simulink model "SecRwLtStLgrstUpwdDnwdTrgtPosSelc"  (R2018b)
settings: Solver=FixedStepDiscrete  StartTime=0.0  StopTime=10.0  FixedStep=0.01  RelTol=1e-3
undefined symbols (not defined in the file or in its folder): KeSMSw4SAcsMd22SecRwLtStLegrstUpwdDnwdPos_Val, KeSMSw4SAcsMd22SecRwLtStLegrstUpwdDnwdPosMax_Val, KeSMSw4SAcsMd22SecRwLtStLegrstUpwdDnwdPosMin_Val, KeSMSw4SAcsMd26SecRwLtStLegrstUpwdDnwdPos_Val, KeSMSw4SAcsMd26SecRwLtStLegrstUpwdDnwdPosMax_Val, KeSMSw4SAcsMd26SecRwLtStLegrstUpwdDnwdPosMin_Val, KeSMSw4SLegrstCloseMdSecRwLtStLgrstUpwdDnwdPos_Val, KeSMSw4SLegrstCloseMdSecRwLtStLgrstUpwdDnwdPosMax_Val, KeSMSw4SLegrstCloseMdSecRwLtStLgrstUpwdDnwdPosMin_Val, KeSMSw4SLegrstOpenMdSecRwLtStLgrstUpwdDnwdPos_Val, KeSMSw4SLegrstOpenMdSecRwLtStLgrstUpwdDnwdPosMax_Val, KeSMSw4SLegrstOpenMdSecRwLtStLgrstUpwdDnwdPosMin_Val, KeSMSw4sLyingMDSecRwLtStLgrstUpwdDnwdPos_Val, KeSMSw4sLyingMDSecRwLtStLgrstUpwdDnwdPosMax_Val, KeSMSw4sLyingMDSecRwLtStLgrstUpwdDnwdPosMin_Val, KeSMSw4sRecoveryMDSecRwLtStLgrstUpwdDnwdPos_Val, KeSMSw4sRecoveryMDSecRwLtStLgrstUpwdDnwdPosMax_Val, KeSMSw4sRecoveryMDSecRwLtStLgrstUpwdDnwdPosMin_Val, KeSMSw4sVIPMDSecRwLtStLgrstUpwdDnwdPos_Val, KeSMSw4sVIPMDSecRwLtStLgrstUpwdDnwdPosMax_Val, KeSMSw4sVIPMDSecRwLtStLgrstUpwdDnwdPosMin_Val, KeSMSw6sAcsEntrySecRwLtStLgrstUpwdPos_Val, KeSMSw6sAcsEntrySecRwLtStLgrstUpwdPosMax_Val, KeSMSw6sAcsEntrySecRwLtStLgrstUpwdPosMin_Val, KeSMSw6sAcsExtSecRwLtStLgrstUpwdDnwdPos_Val, KeSMSw6sAcsExtSecRwLtStLgrstUpwdDnwdPosMax_Val, KeSMSw6sAcsExtSecRwLtStLgrstUpwdDnwdPosMin_Val, KeSMSw6sRecoveryMdSecRwLtStLgrstUpwdDnwdPos_Val, KeSMSw6sRecoveryMdSecRwLtStLgrstUpwdDnwdPosMax_Val, KeSMSw6sRecoveryMdSecRwLtStLgrstUpwdDnwdPosMin_Val, KeSMSw6sVIPSecRwLtStLgrstUpwdPos_Val, KeSMSw6sVIPSecRwLtStLgrstUpwdPosMax_Val, KeSMSw6sVIPSecRwLtStLgrstUpwdPosMin_Val, KeSMSwAcsEntrySecRwLtStLgrstUpwdPos_Val, KeSMSwAcsEntrySecRwLtStLgrstUpwdPosMax_Val, KeSMSwAcsEntrySecRwLtStLgrstUpwdPosMin_Val, KeSMSwAcsExtSecRwLtStLgrstUpwdDnwdPos_Val, KeSMSwAcsExtSecRwLtStLgrstUpwdDnwdPosMax_Val, KeSMSwAcsExtSecRwLtStLgrstUpwdDnwdPosMin_Val, KeSMSwAcsMd8SecRwLtStLgrstUpwdDnwdPos_Val, KeSMSwAcsMd8SecRwLtStLgrstUpwdDnwdPosMax_Val, KeSMSwAcsMd8SecRwLtStLgrstUpwdDnwdPosMin_Val, KeSMSwRecoveryMdSecRwLtStLgrstUpwdDnwdPos_Val, KeSMSwRecoveryMdSecRwLtStLgrstUpwdDnwdPosMax_Val, KeSMSwRecoveryMdSecRwLtStLgrstUpwdDnwdPosMin_Val, KeSMSwVIPSecRwLtStLgrstUpwdPos_Val, KeSMSwVIPSecRwLtStLgrstUpwdPosMax_Val, KeSMSwVIPSecRwLtStLgrstUpwdPosMin_Val
libraries: TrgtPosSelcLib x11
settings Model: Creator=sn2xws  LastModifiedBy=sn2xws
settings Model: ModifiedHistory=|
  | 2023.8.1 V2.0.0 CR401790 增加模式21-26
  | 2024.7.8 V3.0.0 557模式流程V1.9
settings DataIOCC: SaveFormat=StructureWithTime
settings OptimizationCC: DefaultParameterBehavior=Inlined  EnhancedBackFolding=on  PassReuseOutputArgsAs=Individual arguments  ZeroExternalMemoryAtStartup=off  ZeroInternalMemoryAtStartup=off  OptimizeBlockOrder=speed  DifferentSizesBufferReuse=on  OptimizationCustomize=off
settings DebuggingCC: ParameterTunabilityLossMsg=error
settings ModelReferenceCC: ModelReferenceNumInstancesAllowed=Single
settings SFSimCC: MATLABDynamicMemAlloc=off
settings RTWCC: SystemTargetFile=autosar.tlc  GenCodeOnly=on  TemplateMakefile=ert_default_tmf  Description=AUTOSAR  GenerateReport=on  IncludeHyperlinkInReport=on  LaunchReport=on  GenerateTraceInfo=on  GenerateTraceReport=on  GenerateTraceReportSl=on  GenerateTraceReportSf=on  GenerateTraceReportEml=on  GenerateCodeMetricsReport=on
settings CodeAppCC: ForceParamTrailComments=on  IgnoreCustomStorageClasses=off  OperatorAnnotations=on  SimulinkDataObjDesc=on  SFDataObjDesc=on  InsertBlockDesc=on
settings STFCustomTargetCC: TargetLangStandard=C99 (ISO)  MultiwordLength=256  ParMdlRefBuildCompliant=on  CompOptLevelCompliant=on  IncludeMdlTerminateFcn=off  CombineOutputUpdateFcns=on  SuppressErrorStatus=on  ERTCustomFileBanners=on  SupportNonFinite=off  SupportComplex=off  SupportContinuousTime=off  SupportNonInlinedSFcns=off  RemoveResetFunc=on  MATLABClassNameForMDSCustomization=Simulink.SoftwareTarget.ERTCustomization  AutosarCompliant=on  UseToolchainInfoCompliant=on  LookupTableObjectStructAxisOrder=2,1,3,4,...  LUTObjectStructOrderEvenSpacing=Size,Table,Breakpoints  SystemTargetFile=autosar.tlc
settings ERTTargetCC: TargetLangStandard=C99 (ISO)  ConcurrentExecutionCompliant=off  IncludeMdlTerminateFcn=off  SuppressErrorStatus=on  SupportNonFinite=off  SupportComplex=off  ModelStepFunctionPrototypeControlCompliant=off  CPPClassGenCompliant=off  AutosarCompliant=on  LookupTableObjectStructAxisOrder=2,1,3,4,...  LUTObjectStructOrderEvenSpacing=Size,Table,Breakpoints  InlinedParameterPlacement=NonHierarchical  ERTCustomFileTemplate=example_file_process.tlc  ERTFilePackagingFormat=Compact

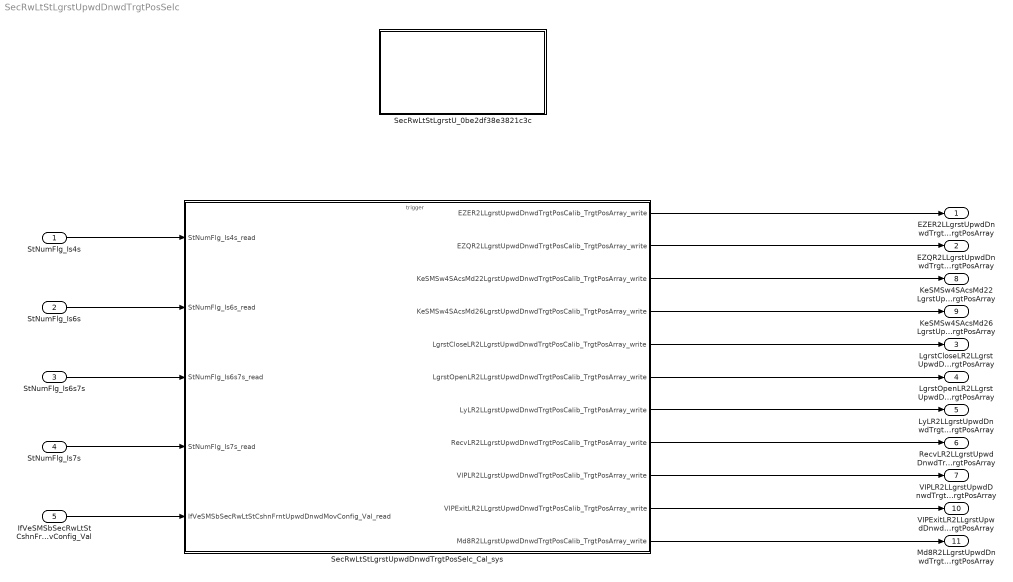
== system SecRwLtStLgrstUpwdDnwdTrgtPosSelc ==
  StNumFlg_Is4s : Inport  OutDataTypeStr=boolean  PortDimensions=1
  StNumFlg_Is6s : Inport  Port=2  OutDataTypeStr=boolean  PortDimensions=1
  StNumFlg_Is6s7s : Inport  Port=3  OutDataTypeStr=boolean  PortDimensions=1
  StNumFlg_Is7s : Inport  Port=4  OutDataTypeStr=boolean  PortDimensions=1
  IfVeSMSbSecRwLtStCshnFrntUpwdDnwdMovConfig_Val : Inport  Port=5  OutDataTypeStr=boolean  PortDimensions=1
  SecRwLtStLgrstU_0be2df38e3821c3c : Subsystem
  SecRwLtStLgrstUpwdDnwdTrgtPosSelc_Cal_sys : Subsystem
  EZER2LLgrstUpwdDnwdTrgtPosCalib_TrgtPosArray : Outport  Description=|  OutDataTypeStr=uint16  PortDimensions=3
      | 0:Pos
      | 1:Max
      | 2:Min
  EZQR2LLgrstUpwdDnwdTrgtPosCalib_TrgtPosArray : Outport  Description=|  Port=2  OutDataTypeStr=uint16  PortDimensions=3
      | 0:Pos
      | 1:Max
      | 2:Min
  LgrstCloseLR2LLgrstUpwdDnwdTrgtPosCalib_TrgtPosArray : Outport  Description=|  Port=3  OutDataTypeStr=uint16  PortDimensions=3
      | 0:Pos
      | 1:Max
      | 2:Min
  LgrstOpenLR2LLgrstUpwdDnwdTrgtPosCalib_TrgtPosArray : Outport  Description=|  Port=4  OutDataTypeStr=uint16  PortDimensions=3
      | 0:Pos
      | 1:Max
      | 2:Min
  LyLR2LLgrstUpwdDnwdTrgtPosCalib_TrgtPosArray : Outport  Description=|  Port=5  OutDataTypeStr=uint16  PortDimensions=3
      | 0:Pos
      | 1:Max
      | 2:Min
  RecvLR2LLgrstUpwdDnwdTrgtPosCalib_TrgtPosArray : Outport  Description=|  Port=6  OutDataTypeStr=uint16  PortDimensions=3
      | 0:Pos
      | 1:Max
      | 2:Min
  VIPLR2LLgrstUpwdDnwdTrgtPosCalib_TrgtPosArray : Outport  Description=|  Port=7  OutDataTypeStr=uint16  PortDimensions=3
      | 0:Pos
      | 1:Max
      | 2:Min
  KeSMSw4SAcsMd22LgrstUpwdDnwdTrgtPosCalib_TrgtPosArray : Outport  Description=|  Port=8  OutDataTypeStr=uint16  PortDimensions=3
      | 0:Pos
      | 1:Max
      | 2:Min
  KeSMSw4SAcsMd26LgrstUpwdDnwdTrgtPosCalib_TrgtPosArray : Outport  Description=|  Port=9  OutDataTypeStr=uint16  PortDimensions=3
      | 0:Pos
      | 1:Max
      | 2:Min
  VIPExitLR2LLgrstUpwdDnwdTrgtPosCalib_TrgtPosArray : Outport  Description=|  Port=10  OutDataTypeStr=uint16  PortDimensions=3
      | 0:Pos
      | 1:Max
      | 2:Min
  Md8R2LLgrstUpwdDnwdTrgtPosCalib_TrgtPosArray : Outport  Description=|  Port=11  OutDataTypeStr=uint16  PortDimensions=3
      | 0:Pos
      | 1:Max
      | 2:Min
  wires:
  StNumFlg_Is4s/1 -> SecRwLtStLgrstUpwdDnwdTrgtPosSelc_Cal_sys/1(StNumFlg_Is4s_read)
  StNumFlg_Is6s/1 -> SecRwLtStLgrstUpwdDnwdTrgtPosSelc_Cal_sys/2(StNumFlg_Is6s_read)
  StNumFlg_Is6s7s/1 -> SecRwLtStLgrstUpwdDnwdTrgtPosSelc_Cal_sys/3(StNumFlg_Is6s7s_read)
  StNumFlg_Is7s/1 -> SecRwLtStLgrstUpwdDnwdTrgtPosSelc_Cal_sys/4(StNumFlg_Is7s_read)
  SecRwLtStLgrstUpwdDnwdTrgtPosSelc_Cal_sys/1(EZER2LLgrstUpwdDnwdTrgtPosCalib_TrgtPosArray_write) -> EZER2LLgrstUpwdDnwdTrgtPosCalib_TrgtPosArray/1
  SecRwLtStLgrstUpwdDnwdTrgtPosSelc_Cal_sys/2(EZQR2LLgrstUpwdDnwdTrgtPosCalib_TrgtPosArray_write) -> EZQR2LLgrstUpwdDnwdTrgtPosCalib_TrgtPosArray/1
  SecRwLtStLgrstUpwdDnwdTrgtPosSelc_Cal_sys/5(LgrstCloseLR2LLgrstUpwdDnwdTrgtPosCalib_TrgtPosArray_write) -> LgrstCloseLR2LLgrstUpwdDnwdTrgtPosCalib_TrgtPosArray/1
  SecRwLtStLgrstUpwdDnwdTrgtPosSelc_Cal_sys/6(LgrstOpenLR2LLgrstUpwdDnwdTrgtPosCalib_TrgtPosArray_write) -> LgrstOpenLR2LLgrstUpwdDnwdTrgtPosCalib_TrgtPosArray/1
  SecRwLtStLgrstUpwdDnwdTrgtPosSelc_Cal_sys/7(LyLR2LLgrstUpwdDnwdTrgtPosCalib_TrgtPosArray_write) -> LyLR2LLgrstUpwdDnwdTrgtPosCalib_TrgtPosArray/1
  SecRwLtStLgrstUpwdDnwdTrgtPosSelc_Cal_sys/8(RecvLR2LLgrstUpwdDnwdTrgtPosCalib_TrgtPosArray_write) -> RecvLR2LLgrstUpwdDnwdTrgtPosCalib_TrgtPosArray/1
  SecRwLtStLgrstUpwdDnwdTrgtPosSelc_Cal_sys/9(VIPLR2LLgrstUpwdDnwdTrgtPosCalib_TrgtPosArray_write) -> VIPLR2LLgrstUpwdDnwdTrgtPosCalib_TrgtPosArray/1
  SecRwLtStLgrstUpwdDnwdTrgtPosSelc_Cal_sys/3(KeSMSw4SAcsMd22LgrstUpwdDnwdTrgtPosCalib_TrgtPosArray_write) -> KeSMSw4SAcsMd22LgrstUpwdDnwdTrgtPosCalib_TrgtPosArray/1
  SecRwLtStLgrstUpwdDnwdTrgtPosSelc_Cal_sys/4(KeSMSw4SAcsMd26LgrstUpwdDnwdTrgtPosCalib_TrgtPosArray_write) -> KeSMSw4SAcsMd26LgrstUpwdDnwdTrgtPosCalib_TrgtPosArray/1
  IfVeSMSbSecRwLtStCshnFrntUpwdDnwdMovConfig_Val/1 -> SecRwLtStLgrstUpwdDnwdTrgtPosSelc_Cal_sys/5(IfVeSMSbSecRwLtStCshnFrntUpwdDnwdMovConfig_Val_read)
  SecRwLtStLgrstUpwdDnwdTrgtPosSelc_Cal_sys/10(VIPExitLR2LLgrstUpwdDnwdTrgtPosCalib_TrgtPosArray_write) -> VIPExitLR2LLgrstUpwdDnwdTrgtPosCalib_TrgtPosArray/1
  SecRwLtStLgrstUpwdDnwdTrgtPosSelc_Cal_sys/11(Md8R2LLgrstUpwdDnwdTrgtPosCalib_TrgtPosArray_write) -> Md8R2LLgrstUpwdDnwdTrgtPosCalib_TrgtPosArray/1

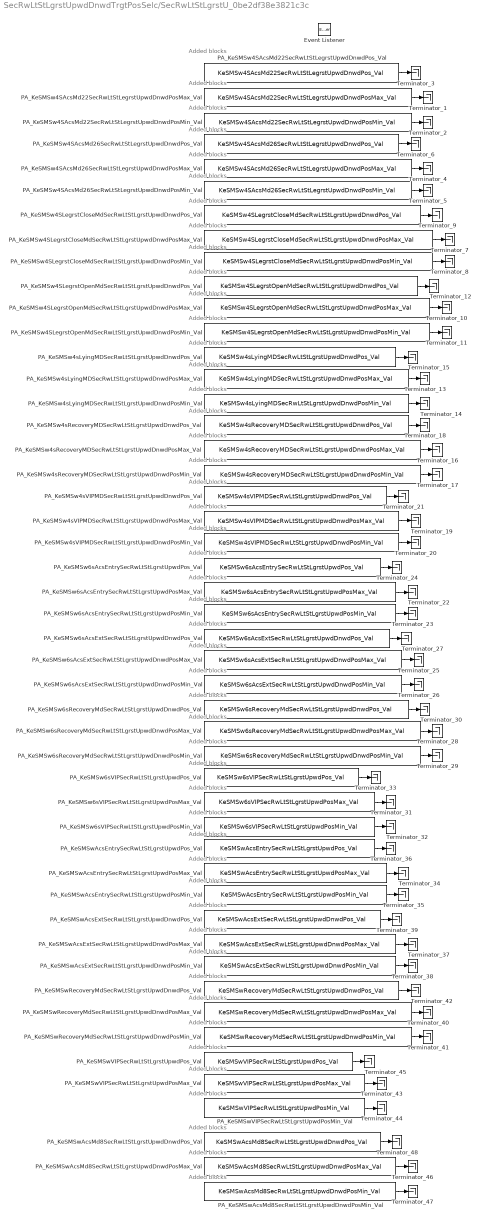
== system SecRwLtStLgrstUpwdDnwdTrgtPosSelc/SecRwLtStLgrstU_0be2df38e3821c3c ==
  note: Added blocks
  note: Added blocks
  note: Added blocks
  note: Added blocks
  note: Added blocks
  note: Added blocks
  note: Added blocks
  note: Added blocks
  note: Added blocks
  note: Added blocks
  note: Added blocks
  note: Added blocks
  note: Added blocks
  note: Added blocks
  note: Added blocks
  note: Added blocks
  note: Added blocks
  note: Added blocks
  note: Added blocks
  note: Added blocks
  note: Added blocks
  note: Added blocks
  note: Added blocks
  note: Added blocks
  note: Added blocks
  note: Added blocks
  note: Added blocks
  note: Added blocks
  note: Added blocks
  note: Added blocks
  note: Added blocks
  note: Added blocks
  note: Added blocks
  note: Added blocks
  note: Added blocks
  note: Added blocks
  note: Added blocks
  note: Added blocks
  note: Added blocks
  note: Added blocks
  note: Added blocks
  note: Added blocks
  note: Added blocks
  note: Added blocks
  note: Added blocks
  note: Added blocks
  note: Added blocks
  note: Added blocks
  Event Listener : EventListener  EventName=reset
  PA_KeSMSw4SAcsMd22SecRwLtStLegrstUpwdDnwdPosMax_Val : Constant  Value=KeSMSw4SAcsMd22SecRwLtStLegrstUpwdDnwdPosMax_Val
  PA_KeSMSw4SAcsMd22SecRwLtStLegrstUpwdDnwdPosMin_Val : Constant  Value=KeSMSw4SAcsMd22SecRwLtStLegrstUpwdDnwdPosMin_Val
  PA_KeSMSw4SAcsMd22SecRwLtStLegrstUpwdDnwdPos_Val : Constant  Value=KeSMSw4SAcsMd22SecRwLtStLegrstUpwdDnwdPos_Val
  PA_KeSMSw4SAcsMd26SecRwLtStLegrstUpwdDnwdPosMax_Val : Constant  Value=KeSMSw4SAcsMd26SecRwLtStLegrstUpwdDnwdPosMax_Val
  PA_KeSMSw4SAcsMd26SecRwLtStLegrstUpwdDnwdPosMin_Val : Constant  Value=KeSMSw4SAcsMd26SecRwLtStLegrstUpwdDnwdPosMin_Val
  PA_KeSMSw4SAcsMd26SecRwLtStLegrstUpwdDnwdPos_Val : Constant  Value=KeSMSw4SAcsMd26SecRwLtStLegrstUpwdDnwdPos_Val
  PA_KeSMSw4SLegrstCloseMdSecRwLtStLgrstUpwdDnwdPosMax_Val : Constant  Value=KeSMSw4SLegrstCloseMdSecRwLtStLgrstUpwdDnwdPosMax_Val
  PA_KeSMSw4SLegrstCloseMdSecRwLtStLgrstUpwdDnwdPosMin_Val : Constant  Value=KeSMSw4SLegrstCloseMdSecRwLtStLgrstUpwdDnwdPosMin_Val
  PA_KeSMSw4SLegrstCloseMdSecRwLtStLgrstUpwdDnwdPos_Val : Constant  Value=KeSMSw4SLegrstCloseMdSecRwLtStLgrstUpwdDnwdPos_Val
  PA_KeSMSw4SLegrstOpenMdSecRwLtStLgrstUpwdDnwdPosMax_Val : Constant  Value=KeSMSw4SLegrstOpenMdSecRwLtStLgrstUpwdDnwdPosMax_Val
  PA_KeSMSw4SLegrstOpenMdSecRwLtStLgrstUpwdDnwdPosMin_Val : Constant  Value=KeSMSw4SLegrstOpenMdSecRwLtStLgrstUpwdDnwdPosMin_Val
  PA_KeSMSw4SLegrstOpenMdSecRwLtStLgrstUpwdDnwdPos_Val : Constant  Value=KeSMSw4SLegrstOpenMdSecRwLtStLgrstUpwdDnwdPos_Val
  PA_KeSMSw4sLyingMDSecRwLtStLgrstUpwdDnwdPosMax_Val : Constant  Value=KeSMSw4sLyingMDSecRwLtStLgrstUpwdDnwdPosMax_Val
  PA_KeSMSw4sLyingMDSecRwLtStLgrstUpwdDnwdPosMin_Val : Constant  Value=KeSMSw4sLyingMDSecRwLtStLgrstUpwdDnwdPosMin_Val
  PA_KeSMSw4sLyingMDSecRwLtStLgrstUpwdDnwdPos_Val : Constant  Value=KeSMSw4sLyingMDSecRwLtStLgrstUpwdDnwdPos_Val
  PA_KeSMSw4sRecoveryMDSecRwLtStLgrstUpwdDnwdPosMax_Val : Constant  Value=KeSMSw4sRecoveryMDSecRwLtStLgrstUpwdDnwdPosMax_Val
  PA_KeSMSw4sRecoveryMDSecRwLtStLgrstUpwdDnwdPosMin_Val : Constant  Value=KeSMSw4sRecoveryMDSecRwLtStLgrstUpwdDnwdPosMin_Val
  PA_KeSMSw4sRecoveryMDSecRwLtStLgrstUpwdDnwdPos_Val : Constant  Value=KeSMSw4sRecoveryMDSecRwLtStLgrstUpwdDnwdPos_Val
  PA_KeSMSw4sVIPMDSecRwLtStLgrstUpwdDnwdPosMax_Val : Constant  Value=KeSMSw4sVIPMDSecRwLtStLgrstUpwdDnwdPosMax_Val
  PA_KeSMSw4sVIPMDSecRwLtStLgrstUpwdDnwdPosMin_Val : Constant  Value=KeSMSw4sVIPMDSecRwLtStLgrstUpwdDnwdPosMin_Val
  PA_KeSMSw4sVIPMDSecRwLtStLgrstUpwdDnwdPos_Val : Constant  Value=KeSMSw4sVIPMDSecRwLtStLgrstUpwdDnwdPos_Val
  PA_KeSMSw6sAcsEntrySecRwLtStLgrstUpwdPosMax_Val : Constant  Value=KeSMSw6sAcsEntrySecRwLtStLgrstUpwdPosMax_Val
  PA_KeSMSw6sAcsEntrySecRwLtStLgrstUpwdPosMin_Val : Constant  Value=KeSMSw6sAcsEntrySecRwLtStLgrstUpwdPosMin_Val
  PA_KeSMSw6sAcsEntrySecRwLtStLgrstUpwdPos_Val : Constant  Value=KeSMSw6sAcsEntrySecRwLtStLgrstUpwdPos_Val
  PA_KeSMSw6sAcsExtSecRwLtStLgrstUpwdDnwdPosMax_Val : Constant  Value=KeSMSw6sAcsExtSecRwLtStLgrstUpwdDnwdPosMax_Val
  PA_KeSMSw6sAcsExtSecRwLtStLgrstUpwdDnwdPosMin_Val : Constant  Value=KeSMSw6sAcsExtSecRwLtStLgrstUpwdDnwdPosMin_Val
  PA_KeSMSw6sAcsExtSecRwLtStLgrstUpwdDnwdPos_Val : Constant  Value=KeSMSw6sAcsExtSecRwLtStLgrstUpwdDnwdPos_Val
  PA_KeSMSw6sRecoveryMdSecRwLtStLgrstUpwdDnwdPosMax_Val : Constant  Value=KeSMSw6sRecoveryMdSecRwLtStLgrstUpwdDnwdPosMax_Val
  PA_KeSMSw6sRecoveryMdSecRwLtStLgrstUpwdDnwdPosMin_Val : Constant  Value=KeSMSw6sRecoveryMdSecRwLtStLgrstUpwdDnwdPosMin_Val
  PA_KeSMSw6sRecoveryMdSecRwLtStLgrstUpwdDnwdPos_Val : Constant  Value=KeSMSw6sRecoveryMdSecRwLtStLgrstUpwdDnwdPos_Val
  PA_KeSMSw6sVIPSecRwLtStLgrstUpwdPosMax_Val : Constant  Value=KeSMSw6sVIPSecRwLtStLgrstUpwdPosMax_Val
  PA_KeSMSw6sVIPSecRwLtStLgrstUpwdPosMin_Val : Constant  Value=KeSMSw6sVIPSecRwLtStLgrstUpwdPosMin_Val
  PA_KeSMSw6sVIPSecRwLtStLgrstUpwdPos_Val : Constant  Value=KeSMSw6sVIPSecRwLtStLgrstUpwdPos_Val
  PA_KeSMSwAcsEntrySecRwLtStLgrstUpwdPosMax_Val : Constant  Value=KeSMSwAcsEntrySecRwLtStLgrstUpwdPosMax_Val
  PA_KeSMSwAcsEntrySecRwLtStLgrstUpwdPosMin_Val : Constant  Value=KeSMSwAcsEntrySecRwLtStLgrstUpwdPosMin_Val
  PA_KeSMSwAcsEntrySecRwLtStLgrstUpwdPos_Val : Constant  Value=KeSMSwAcsEntrySecRwLtStLgrstUpwdPos_Val
  PA_KeSMSwAcsExtSecRwLtStLgrstUpwdDnwdPosMax_Val : Constant  Value=KeSMSwAcsExtSecRwLtStLgrstUpwdDnwdPosMax_Val
  PA_KeSMSwAcsExtSecRwLtStLgrstUpwdDnwdPosMin_Val : Constant  Value=KeSMSwAcsExtSecRwLtStLgrstUpwdDnwdPosMin_Val
  PA_KeSMSwAcsExtSecRwLtStLgrstUpwdDnwdPos_Val : Constant  Value=KeSMSwAcsExtSecRwLtStLgrstUpwdDnwdPos_Val
  PA_KeSMSwAcsMd8SecRwLtStLgrstUpwdDnwdPosMax_Val : Constant  Value=KeSMSwAcsMd8SecRwLtStLgrstUpwdDnwdPosMax_Val
  PA_KeSMSwAcsMd8SecRwLtStLgrstUpwdDnwdPosMin_Val : Constant  Value=KeSMSwAcsMd8SecRwLtStLgrstUpwdDnwdPosMin_Val
  PA_KeSMSwAcsMd8SecRwLtStLgrstUpwdDnwdPos_Val : Constant  Value=KeSMSwAcsMd8SecRwLtStLgrstUpwdDnwdPos_Val
  PA_KeSMSwRecoveryMdSecRwLtStLgrstUpwdDnwdPosMax_Val : Constant  Value=KeSMSwRecoveryMdSecRwLtStLgrstUpwdDnwdPosMax_Val
  PA_KeSMSwRecoveryMdSecRwLtStLgrstUpwdDnwdPosMin_Val : Constant  Value=KeSMSwRecoveryMdSecRwLtStLgrstUpwdDnwdPosMin_Val
  PA_KeSMSwRecoveryMdSecRwLtStLgrstUpwdDnwdPos_Val : Constant  Value=KeSMSwRecoveryMdSecRwLtStLgrstUpwdDnwdPos_Val
  PA_KeSMSwVIPSecRwLtStLgrstUpwdPosMax_Val : Constant  Value=KeSMSwVIPSecRwLtStLgrstUpwdPosMax_Val
  PA_KeSMSwVIPSecRwLtStLgrstUpwdPosMin_Val : Constant  Value=KeSMSwVIPSecRwLtStLgrstUpwdPosMin_Val
  PA_KeSMSwVIPSecRwLtStLgrstUpwdPos_Val : Constant  Value=KeSMSwVIPSecRwLtStLgrstUpwdPos_Val
  Terminator_{1..48} (48 alike) : Terminator
  wires:
  PA_KeSMSw4SAcsMd22SecRwLtStLegrstUpwdDnwdPosMax_Val/1 -> Terminator_1/1
  PA_KeSMSw4SAcsMd22SecRwLtStLegrstUpwdDnwdPosMin_Val/1 -> Terminator_2/1
  PA_KeSMSw4SAcsMd22SecRwLtStLegrstUpwdDnwdPos_Val/1 -> Terminator_3/1
  PA_KeSMSw4SAcsMd26SecRwLtStLegrstUpwdDnwdPosMax_Val/1 -> Terminator_4/1
  PA_KeSMSw4SAcsMd26SecRwLtStLegrstUpwdDnwdPosMin_Val/1 -> Terminator_5/1
  PA_KeSMSw4SAcsMd26SecRwLtStLegrstUpwdDnwdPos_Val/1 -> Terminator_6/1
  PA_KeSMSw4SLegrstCloseMdSecRwLtStLgrstUpwdDnwdPosMax_Val/1 -> Terminator_7/1
  PA_KeSMSw4SLegrstCloseMdSecRwLtStLgrstUpwdDnwdPosMin_Val/1 -> Terminator_8/1
  PA_KeSMSw4SLegrstCloseMdSecRwLtStLgrstUpwdDnwdPos_Val/1 -> Terminator_9/1
  PA_KeSMSw4SLegrstOpenMdSecRwLtStLgrstUpwdDnwdPosMax_Val/1 -> Terminator_10/1
  PA_KeSMSw4SLegrstOpenMdSecRwLtStLgrstUpwdDnwdPosMin_Val/1 -> Terminator_11/1
  PA_KeSMSw4SLegrstOpenMdSecRwLtStLgrstUpwdDnwdPos_Val/1 -> Terminator_12/1
  PA_KeSMSw4sLyingMDSecRwLtStLgrstUpwdDnwdPosMax_Val/1 -> Terminator_13/1
  PA_KeSMSw4sLyingMDSecRwLtStLgrstUpwdDnwdPosMin_Val/1 -> Terminator_14/1
  PA_KeSMSw4sLyingMDSecRwLtStLgrstUpwdDnwdPos_Val/1 -> Terminator_15/1
  PA_KeSMSw4sRecoveryMDSecRwLtStLgrstUpwdDnwdPosMax_Val/1 -> Terminator_16/1
  PA_KeSMSw4sRecoveryMDSecRwLtStLgrstUpwdDnwdPosMin_Val/1 -> Terminator_17/1
  PA_KeSMSw4sRecoveryMDSecRwLtStLgrstUpwdDnwdPos_Val/1 -> Terminator_18/1
  PA_KeSMSw4sVIPMDSecRwLtStLgrstUpwdDnwdPosMax_Val/1 -> Terminator_19/1
  PA_KeSMSw4sVIPMDSecRwLtStLgrstUpwdDnwdPosMin_Val/1 -> Terminator_20/1
  PA_KeSMSw4sVIPMDSecRwLtStLgrstUpwdDnwdPos_Val/1 -> Terminator_21/1
  PA_KeSMSw6sAcsEntrySecRwLtStLgrstUpwdPosMax_Val/1 -> Terminator_22/1
  PA_KeSMSw6sAcsEntrySecRwLtStLgrstUpwdPosMin_Val/1 -> Terminator_23/1
  PA_KeSMSw6sAcsEntrySecRwLtStLgrstUpwdPos_Val/1 -> Terminator_24/1
  PA_KeSMSw6sAcsExtSecRwLtStLgrstUpwdDnwdPosMax_Val/1 -> Terminator_25/1
  PA_KeSMSw6sAcsExtSecRwLtStLgrstUpwdDnwdPosMin_Val/1 -> Terminator_26/1
  PA_KeSMSw6sAcsExtSecRwLtStLgrstUpwdDnwdPos_Val/1 -> Terminator_27/1
  PA_KeSMSw6sRecoveryMdSecRwLtStLgrstUpwdDnwdPosMax_Val/1 -> Terminator_28/1
  PA_KeSMSw6sRecoveryMdSecRwLtStLgrstUpwdDnwdPosMin_Val/1 -> Terminator_29/1
  PA_KeSMSw6sRecoveryMdSecRwLtStLgrstUpwdDnwdPos_Val/1 -> Terminator_30/1
  PA_KeSMSw6sVIPSecRwLtStLgrstUpwdPosMax_Val/1 -> Terminator_31/1
  PA_KeSMSw6sVIPSecRwLtStLgrstUpwdPosMin_Val/1 -> Terminator_32/1
  PA_KeSMSw6sVIPSecRwLtStLgrstUpwdPos_Val/1 -> Terminator_33/1
  PA_KeSMSwAcsEntrySecRwLtStLgrstUpwdPosMax_Val/1 -> Terminator_34/1
  PA_KeSMSwAcsEntrySecRwLtStLgrstUpwdPosMin_Val/1 -> Terminator_35/1
  PA_KeSMSwAcsEntrySecRwLtStLgrstUpwdPos_Val/1 -> Terminator_36/1
  PA_KeSMSwAcsExtSecRwLtStLgrstUpwdDnwdPosMax_Val/1 -> Terminator_37/1
  PA_KeSMSwAcsExtSecRwLtStLgrstUpwdDnwdPosMin_Val/1 -> Terminator_38/1
  PA_KeSMSwAcsExtSecRwLtStLgrstUpwdDnwdPos_Val/1 -> Terminator_39/1
  PA_KeSMSwRecoveryMdSecRwLtStLgrstUpwdDnwdPosMax_Val/1 -> Terminator_40/1
  PA_KeSMSwRecoveryMdSecRwLtStLgrstUpwdDnwdPosMin_Val/1 -> Terminator_41/1
  PA_KeSMSwRecoveryMdSecRwLtStLgrstUpwdDnwdPos_Val/1 -> Terminator_42/1
  PA_KeSMSwVIPSecRwLtStLgrstUpwdPosMax_Val/1 -> Terminator_43/1
  PA_KeSMSwVIPSecRwLtStLgrstUpwdPosMin_Val/1 -> Terminator_44/1
  PA_KeSMSwVIPSecRwLtStLgrstUpwdPos_Val/1 -> Terminator_45/1
  PA_KeSMSwAcsMd8SecRwLtStLgrstUpwdDnwdPosMax_Val/1 -> Terminator_46/1
  PA_KeSMSwAcsMd8SecRwLtStLgrstUpwdDnwdPosMin_Val/1 -> Terminator_47/1
  PA_KeSMSwAcsMd8SecRwLtStLgrstUpwdDnwdPos_Val/1 -> Terminator_48/1

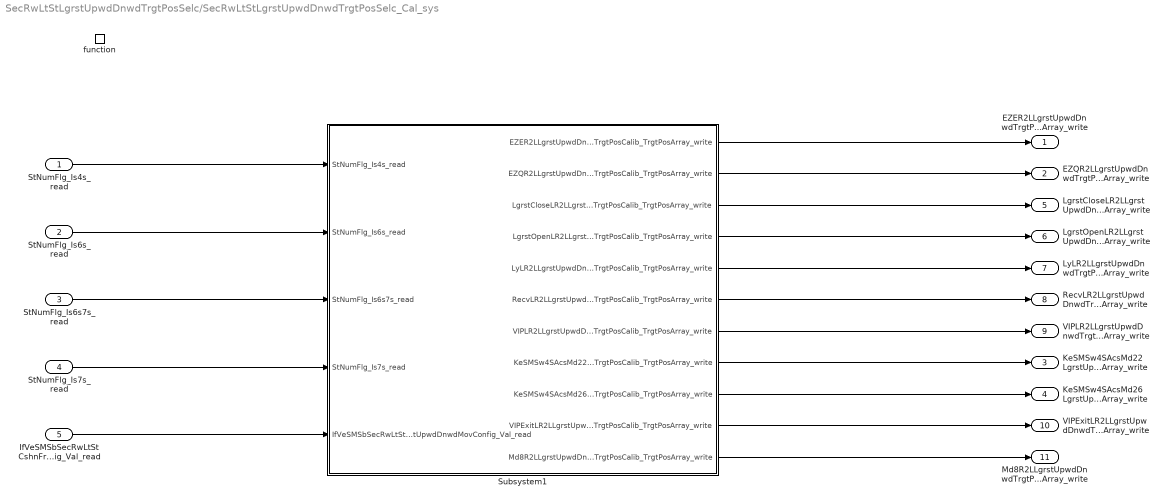
== system SecRwLtStLgrstUpwdDnwdTrgtPosSelc/SecRwLtStLgrstUpwdDnwdTrgtPosSelc_Cal_sys ==
  StNumFlg_Is4s_read : Inport
  StNumFlg_Is6s_read : Inport  Port=2
  StNumFlg_Is6s7s_read : Inport  Port=3
  StNumFlg_Is7s_read : Inport  Port=4
  IfVeSMSbSecRwLtStCshnFrntUpwdDnwdMovConfig_Val_read : Inport  Port=5
  function : TriggerPort  TriggerType=function-call  IsSimulinkFunction=on  FunctionName=SecRwLtStLgrstUpwdDnwdTrgtPosSelc_Cal  VariantControl=(inherit)
  Subsystem1 : Subsystem
  EZER2LLgrstUpwdDnwdTrgtPosCalib_TrgtPosArray_write : Outport
      settings: EnsureOutportIsVirtual=on
  EZQR2LLgrstUpwdDnwdTrgtPosCalib_TrgtPosArray_write : Outport  Port=2
      settings: EnsureOutportIsVirtual=on
  KeSMSw4SAcsMd22LgrstUpwdDnwdTrgtPosCalib_TrgtPosArray_write : Outport  Port=3
      settings: EnsureOutportIsVirtual=on
  KeSMSw4SAcsMd26LgrstUpwdDnwdTrgtPosCalib_TrgtPosArray_write : Outport  Port=4
      settings: EnsureOutportIsVirtual=on
  LgrstCloseLR2LLgrstUpwdDnwdTrgtPosCalib_TrgtPosArray_write : Outport  Port=5
      settings: EnsureOutportIsVirtual=on
  LgrstOpenLR2LLgrstUpwdDnwdTrgtPosCalib_TrgtPosArray_write : Outport  Port=6
      settings: EnsureOutportIsVirtual=on
  LyLR2LLgrstUpwdDnwdTrgtPosCalib_TrgtPosArray_write : Outport  Port=7
      settings: EnsureOutportIsVirtual=on
  RecvLR2LLgrstUpwdDnwdTrgtPosCalib_TrgtPosArray_write : Outport  Port=8
      settings: EnsureOutportIsVirtual=on
  VIPLR2LLgrstUpwdDnwdTrgtPosCalib_TrgtPosArray_write : Outport  Port=9
      settings: EnsureOutportIsVirtual=on
  VIPExitLR2LLgrstUpwdDnwdTrgtPosCalib_TrgtPosArray_write : Outport  Port=10
      settings: EnsureOutportIsVirtual=on
  Md8R2LLgrstUpwdDnwdTrgtPosCalib_TrgtPosArray_write : Outport  Port=11
      settings: EnsureOutportIsVirtual=on
  wires:
  Subsystem1/3(LgrstCloseLR2LLgrstUpwdDnwdTrgtPosCalib_TrgtPosArray_write) -> LgrstCloseLR2LLgrstUpwdDnwdTrgtPosCalib_TrgtPosArray_write/1
  Subsystem1/4(LgrstOpenLR2LLgrstUpwdDnwdTrgtPosCalib_TrgtPosArray_write) -> LgrstOpenLR2LLgrstUpwdDnwdTrgtPosCalib_TrgtPosArray_write/1
  Subsystem1/5(LyLR2LLgrstUpwdDnwdTrgtPosCalib_TrgtPosArray_write) -> LyLR2LLgrstUpwdDnwdTrgtPosCalib_TrgtPosArray_write/1
  Subsystem1/6(RecvLR2LLgrstUpwdDnwdTrgtPosCalib_TrgtPosArray_write) -> RecvLR2LLgrstUpwdDnwdTrgtPosCalib_TrgtPosArray_write/1
  Subsystem1/7(VIPLR2LLgrstUpwdDnwdTrgtPosCalib_TrgtPosArray_write) -> VIPLR2LLgrstUpwdDnwdTrgtPosCalib_TrgtPosArray_write/1
  Subsystem1/1(EZER2LLgrstUpwdDnwdTrgtPosCalib_TrgtPosArray_write) -> EZER2LLgrstUpwdDnwdTrgtPosCalib_TrgtPosArray_write/1
  Subsystem1/2(EZQR2LLgrstUpwdDnwdTrgtPosCalib_TrgtPosArray_write) -> EZQR2LLgrstUpwdDnwdTrgtPosCalib_TrgtPosArray_write/1
  Subsystem1/8(KeSMSw4SAcsMd22LgrstUpwdDnwdTrgtPosCalib_TrgtPosArray_write) -> KeSMSw4SAcsMd22LgrstUpwdDnwdTrgtPosCalib_TrgtPosArray_write/1
  Subsystem1/9(KeSMSw4SAcsMd26LgrstUpwdDnwdTrgtPosCalib_TrgtPosArray_write) -> KeSMSw4SAcsMd26LgrstUpwdDnwdTrgtPosCalib_TrgtPosArray_write/1
  StNumFlg_Is4s_read/1 -> Subsystem1/1(StNumFlg_Is4s_read)
  StNumFlg_Is6s_read/1 -> Subsystem1/2(StNumFlg_Is6s_read)
  StNumFlg_Is6s7s_read/1 -> Subsystem1/3(StNumFlg_Is6s7s_read)
  StNumFlg_Is7s_read/1 -> Subsystem1/4(StNumFlg_Is7s_read)
  IfVeSMSbSecRwLtStCshnFrntUpwdDnwdMovConfig_Val_read/1 -> Subsystem1/5(IfVeSMSbSecRwLtStCshnFrntUpwdDnwdMovConfig_Val_read)
  Subsystem1/10(VIPExitLR2LLgrstUpwdDnwdTrgtPosCalib_TrgtPosArray_write) -> VIPExitLR2LLgrstUpwdDnwdTrgtPosCalib_TrgtPosArray_write/1
  Subsystem1/11(Md8R2LLgrstUpwdDnwdTrgtPosCalib_TrgtPosArray_write) -> Md8R2LLgrstUpwdDnwdTrgtPosCalib_TrgtPosArray_write/1

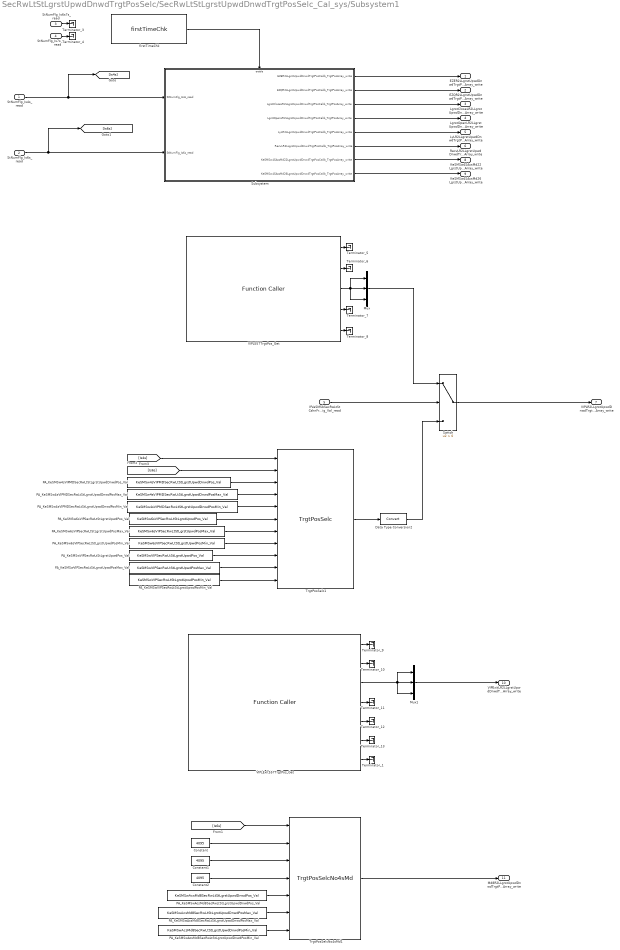
== system SecRwLtStLgrstUpwdDnwdTrgtPosSelc/SecRwLtStLgrstUpwdDnwdTrgtPosSelc_Cal_sys/Subsystem1 ==
  StNumFlg_Is4s_read : Inport
  StNumFlg_Is6s_read : Inport  Port=2
  StNumFlg_Is6s7s_read : Inport  Port=3
  StNumFlg_Is7s_read : Inport  Port=4
  IfVeSMSbSecRwLtStCshnFrntUpwdDnwdMovConfig_Val_read : Inport  Port=5
  Constant : Constant  Value=4095  OutDataTypeStr=uint16
  Constant1 : Constant  Value=4095  OutDataTypeStr=uint16
  Constant2 : Constant  Value=4095  OutDataTypeStr=uint16
  Data Type Conversion2 : DataTypeConversion
  Mux : Mux  Inputs=3
  Mux1 : Mux  Inputs=3
  PA_KeSMSw4sVIPMDSecRwLtStLgrstUpwdDnwdPosMax_Val : Constant  Value=KeSMSw4sVIPMDSecRwLtStLgrstUpwdDnwdPosMax_Val
  PA_KeSMSw4sVIPMDSecRwLtStLgrstUpwdDnwdPosMin_Val : Constant  Value=KeSMSw4sVIPMDSecRwLtStLgrstUpwdDnwdPosMin_Val
  PA_KeSMSw4sVIPMDSecRwLtStLgrstUpwdDnwdPos_Val : Constant  Value=KeSMSw4sVIPMDSecRwLtStLgrstUpwdDnwdPos_Val
  PA_KeSMSw6sVIPSecRwLtStLgrstUpwdPosMax_Val : Constant  Value=KeSMSw6sVIPSecRwLtStLgrstUpwdPosMax_Val
  PA_KeSMSw6sVIPSecRwLtStLgrstUpwdPosMin_Val : Constant  Value=KeSMSw6sVIPSecRwLtStLgrstUpwdPosMin_Val
  PA_KeSMSw6sVIPSecRwLtStLgrstUpwdPos_Val : Constant  Value=KeSMSw6sVIPSecRwLtStLgrstUpwdPos_Val
  PA_KeSMSwAcsMd8SecRwLtStLgrstUpwdDnwdPosMax_Val : Constant  Value=KeSMSwAcsMd8SecRwLtStLgrstUpwdDnwdPosMax_Val
  PA_KeSMSwAcsMd8SecRwLtStLgrstUpwdDnwdPosMin_Val : Constant  Value=KeSMSwAcsMd8SecRwLtStLgrstUpwdDnwdPosMin_Val
  PA_KeSMSwAcsMd8SecRwLtStLgrstUpwdDnwdPos_Val : Constant  Value=KeSMSwAcsMd8SecRwLtStLgrstUpwdDnwdPos_Val
  PA_KeSMSwVIPSecRwLtStLgrstUpwdPosMax_Val : Constant  Value=KeSMSwVIPSecRwLtStLgrstUpwdPosMax_Val
  PA_KeSMSwVIPSecRwLtStLgrstUpwdPosMin_Val : Constant  Value=KeSMSwVIPSecRwLtStLgrstUpwdPosMin_Val
  PA_KeSMSwVIPSecRwLtStLgrstUpwdPos_Val : Constant  Value=KeSMSwVIPSecRwLtStLgrstUpwdPos_Val
  Subsystem : Subsystem
  Switch : Switch  Criteria=u2 > Threshold
  Terminator_{1,3..13} (12 alike) : Terminator
  TrgtPosSelc1 : TrgtPosSelcLib/TrgtPosSelc  SystemSampleTime=-1
  TrgtPosSelcNo4sMd1 : TrgtPosSelcLib/TrgtPosSelcNo4sMd  SystemSampleTime=-1
  VIPL557TrgtPos_Get : FunctionCaller  FunctionPrototype=[SecRwLtStBkReclnTrgtPos,SecRwLtStZeroTrgtPos,SecRwLtStLgrstUpwdDnwdTrgtPos,SecRwLtStLgrstInwdOtwdTrgtPos,SecRwLtStFwdBkwdTrgtPos] = VIPL557TrgtPos_Get()  OutputArgumentSpecifications=uint16(1), uint16(1), uint16(1), uint16(1), uint16(1)
  VIPLExit557TrgtPos_Get : FunctionCaller  FunctionPrototype=[SecRwLtStBkReclnTrgtPos,SecRwLtStZeroTrgtPos,SecRwLtStLgrstUpwdDnwdTrgtPos,SecRwLtStLgrstInwdOtwdTrgtPos,ThdRwLtStBkReclnTrgtPos,ThdRwLtStFwdBkwdTrgtPos,SecRwLtStFwdBkwdTrgtPos] = VIPLExit557TrgtPos_Get()  OutputArgumentSpecifications=uint16(1), uint16(1), uint16(1), uint16(1), uint16(1), uint16(1), uint16(1)
  firstTimeChk : TrgtPosSelcLib/firstTimeChk  SystemSampleTime=-1
  EZER2LLgrstUpwdDnwdTrgtPosCalib_TrgtPosArray_write : Outport
      settings: EnsureOutportIsVirtual=on
  EZQR2LLgrstUpwdDnwdTrgtPosCalib_TrgtPosArray_write : Outport  Port=2
      settings: EnsureOutportIsVirtual=on
  LgrstCloseLR2LLgrstUpwdDnwdTrgtPosCalib_TrgtPosArray_write : Outport  Port=3
      settings: EnsureOutportIsVirtual=on
  LgrstOpenLR2LLgrstUpwdDnwdTrgtPosCalib_TrgtPosArray_write : Outport  Port=4
      settings: EnsureOutportIsVirtual=on
  LyLR2LLgrstUpwdDnwdTrgtPosCalib_TrgtPosArray_write : Outport  Port=5
      settings: EnsureOutportIsVirtual=on
  RecvLR2LLgrstUpwdDnwdTrgtPosCalib_TrgtPosArray_write : Outport  Port=6
      settings: EnsureOutportIsVirtual=on
  VIPLR2LLgrstUpwdDnwdTrgtPosCalib_TrgtPosArray_write : Outport  Port=7
      settings: EnsureOutportIsVirtual=on
  KeSMSw4SAcsMd22LgrstUpwdDnwdTrgtPosCalib_TrgtPosArray_write : Outport  Port=8
      settings: EnsureOutportIsVirtual=on
  KeSMSw4SAcsMd26LgrstUpwdDnwdTrgtPosCalib_TrgtPosArray_write : Outport  Port=9
      settings: EnsureOutportIsVirtual=on
  VIPExitLR2LLgrstUpwdDnwdTrgtPosCalib_TrgtPosArray_write : Outport  Port=10
      settings: EnsureOutportIsVirtual=on
  Md8R2LLgrstUpwdDnwdTrgtPosCalib_TrgtPosArray_write : Outport  Port=11
      settings: EnsureOutportIsVirtual=on
  wires:
  Subsystem/6(RecvLR2LLgrstUpwdDnwdTrgtPosCalib_TrgtPosArray_write) -> RecvLR2LLgrstUpwdDnwdTrgtPosCalib_TrgtPosArray_write/1
  Subsystem/4(LgrstOpenLR2LLgrstUpwdDnwdTrgtPosCalib_TrgtPosArray_write) -> LgrstOpenLR2LLgrstUpwdDnwdTrgtPosCalib_TrgtPosArray_write/1
  StNumFlg_Is6s_read/1 -> [Is6s], Subsystem/2(StNumFlg_Is6s_read)
  firstTimeChk/1 -> Subsystem/Enable
  Subsystem/3(LgrstCloseLR2LLgrstUpwdDnwdTrgtPosCalib_TrgtPosArray_write) -> LgrstCloseLR2LLgrstUpwdDnwdTrgtPosCalib_TrgtPosArray_write/1
  Subsystem/2(EZQR2LLgrstUpwdDnwdTrgtPosCalib_TrgtPosArray_write) -> EZQR2LLgrstUpwdDnwdTrgtPosCalib_TrgtPosArray_write/1
  StNumFlg_Is6s7s_read/1 -> Terminator_3/1
  Subsystem/5(LyLR2LLgrstUpwdDnwdTrgtPosCalib_TrgtPosArray_write) -> LyLR2LLgrstUpwdDnwdTrgtPosCalib_TrgtPosArray_write/1
  Subsystem/1(EZER2LLgrstUpwdDnwdTrgtPosCalib_TrgtPosArray_write) -> EZER2LLgrstUpwdDnwdTrgtPosCalib_TrgtPosArray_write/1
  StNumFlg_Is7s_read/1 -> Terminator_4/1
  StNumFlg_Is4s_read/1 -> [Is4s], Subsystem/1(StNumFlg_Is4s_read)
  Subsystem/7(KeSMSw4SAcsMd22LgrstUpwdDnwdTrgtPosCalib_TrgtPosArray_write) -> KeSMSw4SAcsMd22LgrstUpwdDnwdTrgtPosCalib_TrgtPosArray_write/1
  Subsystem/8(KeSMSw4SAcsMd26LgrstUpwdDnwdTrgtPosCalib_TrgtPosArray_write) -> KeSMSw4SAcsMd26LgrstUpwdDnwdTrgtPosCalib_TrgtPosArray_write/1
  PA_KeSMSwVIPSecRwLtStLgrstUpwdPos_Val/1 -> TrgtPosSelc1/9
  PA_KeSMSw4sVIPMDSecRwLtStLgrstUpwdDnwdPosMin_Val/1 -> TrgtPosSelc1/5
  PA_KeSMSwVIPSecRwLtStLgrstUpwdPosMin_Val/1 -> TrgtPosSelc1/11
  PA_KeSMSw6sVIPSecRwLtStLgrstUpwdPosMin_Val/1 -> TrgtPosSelc1/8
  PA_KeSMSw6sVIPSecRwLtStLgrstUpwdPosMax_Val/1 -> TrgtPosSelc1/7
  PA_KeSMSw4sVIPMDSecRwLtStLgrstUpwdDnwdPosMax_Val/1 -> TrgtPosSelc1/4
  PA_KeSMSw4sVIPMDSecRwLtStLgrstUpwdDnwdPos_Val/1 -> TrgtPosSelc1/3
  TrgtPosSelc1/1 -> Data Type Conversion2/1
  [Is4s] -> TrgtPosSelc1/1
  PA_KeSMSwVIPSecRwLtStLgrstUpwdPosMax_Val/1 -> TrgtPosSelc1/10
  PA_KeSMSw6sVIPSecRwLtStLgrstUpwdPos_Val/1 -> TrgtPosSelc1/6
  [Is6s] -> TrgtPosSelc1/2
  IfVeSMSbSecRwLtStCshnFrntUpwdDnwdMovConfig_Val_read/1 -> Switch/2
  Data Type Conversion2/1 -> Switch/3
  Switch/1 -> VIPLR2LLgrstUpwdDnwdTrgtPosCalib_TrgtPosArray_write/1
  Mux/1 -> Switch/1
  VIPL557TrgtPos_Get/3 -> Mux/3, Mux/1, Mux/2
  VIPLExit557TrgtPos_Get/3 -> Mux1/3, Mux1/1, Mux1/2
  Mux1/1 -> VIPExitLR2LLgrstUpwdDnwdTrgtPosCalib_TrgtPosArray_write/1
  VIPL557TrgtPos_Get/1 -> Terminator_5/1
  VIPL557TrgtPos_Get/2 -> Terminator_6/1
  VIPL557TrgtPos_Get/4 -> Terminator_7/1
  VIPL557TrgtPos_Get/5 -> Terminator_8/1
  VIPLExit557TrgtPos_Get/1 -> Terminator_9/1
  VIPLExit557TrgtPos_Get/2 -> Terminator_10/1
  VIPLExit557TrgtPos_Get/4 -> Terminator_11/1
  VIPLExit557TrgtPos_Get/5 -> Terminator_12/1
  VIPLExit557TrgtPos_Get/6 -> Terminator_13/1
  VIPLExit557TrgtPos_Get/7 -> Terminator_1/1
  TrgtPosSelcNo4sMd1/1 -> Md8R2LLgrstUpwdDnwdTrgtPosCalib_TrgtPosArray_write/1
  [Is6s] -> TrgtPosSelcNo4sMd1/1
  PA_KeSMSwAcsMd8SecRwLtStLgrstUpwdDnwdPosMin_Val/1 -> TrgtPosSelcNo4sMd1/7
  PA_KeSMSwAcsMd8SecRwLtStLgrstUpwdDnwdPosMax_Val/1 -> TrgtPosSelcNo4sMd1/6
  PA_KeSMSwAcsMd8SecRwLtStLgrstUpwdDnwdPos_Val/1 -> TrgtPosSelcNo4sMd1/5
  Constant/1 -> TrgtPosSelcNo4sMd1/2
  Constant1/1 -> TrgtPosSelcNo4sMd1/3
  Constant2/1 -> TrgtPosSelcNo4sMd1/4

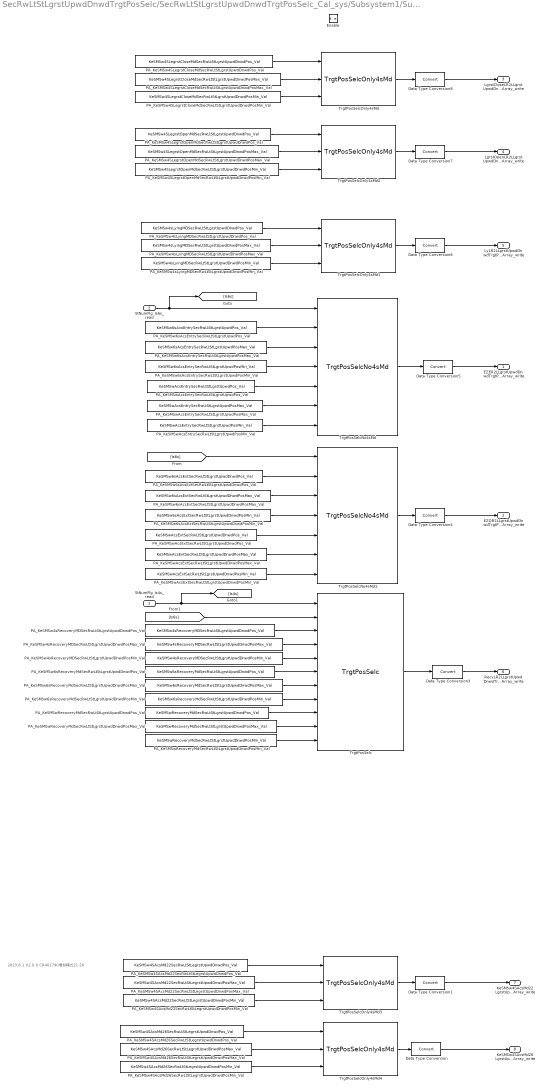
== system SecRwLtStLgrstUpwdDnwdTrgtPosSelc/SecRwLtStLgrstUpwdDnwdTrgtPosSelc_Cal_sys/Subsystem1/Subsystem ==
  note: 2023.8.1 V2.0.0 CR401790 增加模式21-26
  StNumFlg_Is4s_read : Inport
  StNumFlg_Is6s_read : Inport  Port=2
  Enable : EnablePort
  Data Type Conversion{,1,3..8} (8 alike) : DataTypeConversion
  PA_KeSMSw4SAcsMd22SecRwLtStLegrstUpwdDnwdPosMax_Val : Constant  Value=KeSMSw4SAcsMd22SecRwLtStLegrstUpwdDnwdPosMax_Val
  PA_KeSMSw4SAcsMd22SecRwLtStLegrstUpwdDnwdPosMin_Val : Constant  Value=KeSMSw4SAcsMd22SecRwLtStLegrstUpwdDnwdPosMin_Val
  PA_KeSMSw4SAcsMd22SecRwLtStLegrstUpwdDnwdPos_Val : Constant  Value=KeSMSw4SAcsMd22SecRwLtStLegrstUpwdDnwdPos_Val
  PA_KeSMSw4SAcsMd26SecRwLtStLegrstUpwdDnwdPosMax_Val : Constant  Value=KeSMSw4SAcsMd26SecRwLtStLegrstUpwdDnwdPosMax_Val
  PA_KeSMSw4SAcsMd26SecRwLtStLegrstUpwdDnwdPosMin_Val : Constant  Value=KeSMSw4SAcsMd26SecRwLtStLegrstUpwdDnwdPosMin_Val
  PA_KeSMSw4SAcsMd26SecRwLtStLegrstUpwdDnwdPos_Val : Constant  Value=KeSMSw4SAcsMd26SecRwLtStLegrstUpwdDnwdPos_Val
  PA_KeSMSw4SLegrstCloseMdSecRwLtStLgrstUpwdDnwdPosMax_Val : Constant  Value=KeSMSw4SLegrstCloseMdSecRwLtStLgrstUpwdDnwdPosMax_Val
  PA_KeSMSw4SLegrstCloseMdSecRwLtStLgrstUpwdDnwdPosMin_Val : Constant  Value=KeSMSw4SLegrstCloseMdSecRwLtStLgrstUpwdDnwdPosMin_Val
  PA_KeSMSw4SLegrstCloseMdSecRwLtStLgrstUpwdDnwdPos_Val : Constant  Value=KeSMSw4SLegrstCloseMdSecRwLtStLgrstUpwdDnwdPos_Val
  PA_KeSMSw4SLegrstOpenMdSecRwLtStLgrstUpwdDnwdPosMax_Val : Constant  Value=KeSMSw4SLegrstOpenMdSecRwLtStLgrstUpwdDnwdPosMax_Val
  PA_KeSMSw4SLegrstOpenMdSecRwLtStLgrstUpwdDnwdPosMin_Val : Constant  Value=KeSMSw4SLegrstOpenMdSecRwLtStLgrstUpwdDnwdPosMin_Val
  PA_KeSMSw4SLegrstOpenMdSecRwLtStLgrstUpwdDnwdPos_Val : Constant  Value=KeSMSw4SLegrstOpenMdSecRwLtStLgrstUpwdDnwdPos_Val
  PA_KeSMSw4sLyingMDSecRwLtStLgrstUpwdDnwdPosMax_Val : Constant  Value=KeSMSw4sLyingMDSecRwLtStLgrstUpwdDnwdPosMax_Val
  PA_KeSMSw4sLyingMDSecRwLtStLgrstUpwdDnwdPosMin_Val : Constant  Value=KeSMSw4sLyingMDSecRwLtStLgrstUpwdDnwdPosMin_Val
  PA_KeSMSw4sLyingMDSecRwLtStLgrstUpwdDnwdPos_Val : Constant  Value=KeSMSw4sLyingMDSecRwLtStLgrstUpwdDnwdPos_Val
  PA_KeSMSw4sRecoveryMDSecRwLtStLgrstUpwdDnwdPosMax_Val : Constant  Value=KeSMSw4sRecoveryMDSecRwLtStLgrstUpwdDnwdPosMax_Val
  PA_KeSMSw4sRecoveryMDSecRwLtStLgrstUpwdDnwdPosMin_Val : Constant  Value=KeSMSw4sRecoveryMDSecRwLtStLgrstUpwdDnwdPosMin_Val
  PA_KeSMSw4sRecoveryMDSecRwLtStLgrstUpwdDnwdPos_Val : Constant  Value=KeSMSw4sRecoveryMDSecRwLtStLgrstUpwdDnwdPos_Val
  PA_KeSMSw6sAcsEntrySecRwLtStLgrstUpwdPosMax_Val : Constant  Value=KeSMSw6sAcsEntrySecRwLtStLgrstUpwdPosMax_Val
  PA_KeSMSw6sAcsEntrySecRwLtStLgrstUpwdPosMin_Val : Constant  Value=KeSMSw6sAcsEntrySecRwLtStLgrstUpwdPosMin_Val
  PA_KeSMSw6sAcsEntrySecRwLtStLgrstUpwdPos_Val : Constant  Value=KeSMSw6sAcsEntrySecRwLtStLgrstUpwdPos_Val
  PA_KeSMSw6sAcsExtSecRwLtStLgrstUpwdDnwdPosMax_Val : Constant  Value=KeSMSw6sAcsExtSecRwLtStLgrstUpwdDnwdPosMax_Val
  PA_KeSMSw6sAcsExtSecRwLtStLgrstUpwdDnwdPosMin_Val : Constant  Value=KeSMSw6sAcsExtSecRwLtStLgrstUpwdDnwdPosMin_Val
  PA_KeSMSw6sAcsExtSecRwLtStLgrstUpwdDnwdPos_Val : Constant  Value=KeSMSw6sAcsExtSecRwLtStLgrstUpwdDnwdPos_Val
  PA_KeSMSw6sRecoveryMdSecRwLtStLgrstUpwdDnwdPosMax_Val : Constant  Value=KeSMSw6sRecoveryMdSecRwLtStLgrstUpwdDnwdPosMax_Val
  PA_KeSMSw6sRecoveryMdSecRwLtStLgrstUpwdDnwdPosMin_Val : Constant  Value=KeSMSw6sRecoveryMdSecRwLtStLgrstUpwdDnwdPosMin_Val
  PA_KeSMSw6sRecoveryMdSecRwLtStLgrstUpwdDnwdPos_Val : Constant  Value=KeSMSw6sRecoveryMdSecRwLtStLgrstUpwdDnwdPos_Val
  PA_KeSMSwAcsEntrySecRwLtStLgrstUpwdPosMax_Val : Constant  Value=KeSMSwAcsEntrySecRwLtStLgrstUpwdPosMax_Val
  PA_KeSMSwAcsEntrySecRwLtStLgrstUpwdPosMin_Val : Constant  Value=KeSMSwAcsEntrySecRwLtStLgrstUpwdPosMin_Val
  PA_KeSMSwAcsEntrySecRwLtStLgrstUpwdPos_Val : Constant  Value=KeSMSwAcsEntrySecRwLtStLgrstUpwdPos_Val
  PA_KeSMSwAcsExtSecRwLtStLgrstUpwdDnwdPosMax_Val : Constant  Value=KeSMSwAcsExtSecRwLtStLgrstUpwdDnwdPosMax_Val
  PA_KeSMSwAcsExtSecRwLtStLgrstUpwdDnwdPosMin_Val : Constant  Value=KeSMSwAcsExtSecRwLtStLgrstUpwdDnwdPosMin_Val
  PA_KeSMSwAcsExtSecRwLtStLgrstUpwdDnwdPos_Val : Constant  Value=KeSMSwAcsExtSecRwLtStLgrstUpwdDnwdPos_Val
  PA_KeSMSwRecoveryMdSecRwLtStLgrstUpwdDnwdPosMax_Val : Constant  Value=KeSMSwRecoveryMdSecRwLtStLgrstUpwdDnwdPosMax_Val
  PA_KeSMSwRecoveryMdSecRwLtStLgrstUpwdDnwdPosMin_Val : Constant  Value=KeSMSwRecoveryMdSecRwLtStLgrstUpwdDnwdPosMin_Val
  PA_KeSMSwRecoveryMdSecRwLtStLgrstUpwdDnwdPos_Val : Constant  Value=KeSMSwRecoveryMdSecRwLtStLgrstUpwdDnwdPos_Val
  TrgtPosSelc : TrgtPosSelcLib/TrgtPosSelc  SystemSampleTime=-1
  TrgtPosSelcNo4sMd : TrgtPosSelcLib/TrgtPosSelcNo4sMd  SystemSampleTime=-1
  TrgtPosSelcNo4sMd1 : TrgtPosSelcLib/TrgtPosSelcNo4sMd  SystemSampleTime=-1
  TrgtPosSelcOnly4sMd{,1..4} (5 alike) : TrgtPosSelcLib/TrgtPosSelcOnly4sMd  SystemSampleTime=-1
  EZER2LLgrstUpwdDnwdTrgtPosCalib_TrgtPosArray_write : Outport
  EZQR2LLgrstUpwdDnwdTrgtPosCalib_TrgtPosArray_write : Outport  Port=2
  LgrstCloseLR2LLgrstUpwdDnwdTrgtPosCalib_TrgtPosArray_write : Outport  Port=3
  LgrstOpenLR2LLgrstUpwdDnwdTrgtPosCalib_TrgtPosArray_write : Outport  Port=4
  LyLR2LLgrstUpwdDnwdTrgtPosCalib_TrgtPosArray_write : Outport  Port=5
  RecvLR2LLgrstUpwdDnwdTrgtPosCalib_TrgtPosArray_write : Outport  Port=6
  KeSMSw4SAcsMd22LgrstUpwdDnwdTrgtPosCalib_TrgtPosArray_write : Outport  Port=7
  KeSMSw4SAcsMd26LgrstUpwdDnwdTrgtPosCalib_TrgtPosArray_write : Outport  Port=8
  wires:
  PA_KeSMSw6sRecoveryMdSecRwLtStLgrstUpwdDnwdPos_Val/1 -> TrgtPosSelc/6
  [Is6s] -> TrgtPosSelcNo4sMd1/1
  [Is6s] -> TrgtPosSelc/2
  PA_KeSMSw6sAcsExtSecRwLtStLgrstUpwdDnwdPosMin_Val/1 -> TrgtPosSelcNo4sMd1/4
  TrgtPosSelcNo4sMd1/1 -> Data Type Conversion4/1
  PA_KeSMSwAcsExtSecRwLtStLgrstUpwdDnwdPosMax_Val/1 -> TrgtPosSelcNo4sMd1/6
  PA_KeSMSw4SLegrstOpenMdSecRwLtStLgrstUpwdDnwdPosMin_Val/1 -> TrgtPosSelcOnly4sMd2/3
  PA_KeSMSw6sAcsExtSecRwLtStLgrstUpwdDnwdPos_Val/1 -> TrgtPosSelcNo4sMd1/2
  StNumFlg_Is4s_read/1 -> [Is4s], TrgtPosSelc/1
  PA_KeSMSw6sAcsExtSecRwLtStLgrstUpwdDnwdPosMax_Val/1 -> TrgtPosSelcNo4sMd1/3
  PA_KeSMSwAcsExtSecRwLtStLgrstUpwdDnwdPos_Val/1 -> TrgtPosSelcNo4sMd1/5
  PA_KeSMSwAcsExtSecRwLtStLgrstUpwdDnwdPosMin_Val/1 -> TrgtPosSelcNo4sMd1/7
  PA_KeSMSw4sRecoveryMDSecRwLtStLgrstUpwdDnwdPosMax_Val/1 -> TrgtPosSelc/4
  TrgtPosSelcOnly4sMd/1 -> Data Type Conversion8/1
  PA_KeSMSw4sRecoveryMDSecRwLtStLgrstUpwdDnwdPosMin_Val/1 -> TrgtPosSelc/5
  PA_KeSMSw4sRecoveryMDSecRwLtStLgrstUpwdDnwdPos_Val/1 -> TrgtPosSelc/3
  TrgtPosSelcNo4sMd/1 -> Data Type Conversion5/1
  PA_KeSMSw4SLegrstCloseMdSecRwLtStLgrstUpwdDnwdPosMax_Val/1 -> TrgtPosSelcOnly4sMd/2
  PA_KeSMSw6sAcsEntrySecRwLtStLgrstUpwdPosMin_Val/1 -> TrgtPosSelcNo4sMd/4
  PA_KeSMSw4sLyingMDSecRwLtStLgrstUpwdDnwdPosMax_Val/1 -> TrgtPosSelcOnly4sMd1/2
  PA_KeSMSw4SLegrstCloseMdSecRwLtStLgrstUpwdDnwdPosMin_Val/1 -> TrgtPosSelcOnly4sMd/3
  PA_KeSMSw4sLyingMDSecRwLtStLgrstUpwdDnwdPosMin_Val/1 -> TrgtPosSelcOnly4sMd1/3
  PA_KeSMSw6sAcsEntrySecRwLtStLgrstUpwdPosMax_Val/1 -> TrgtPosSelcNo4sMd/3
  PA_KeSMSw6sRecoveryMdSecRwLtStLgrstUpwdDnwdPosMax_Val/1 -> TrgtPosSelc/7
  PA_KeSMSwAcsEntrySecRwLtStLgrstUpwdPosMin_Val/1 -> TrgtPosSelcNo4sMd/7
  PA_KeSMSwAcsEntrySecRwLtStLgrstUpwdPosMax_Val/1 -> TrgtPosSelcNo4sMd/6
  PA_KeSMSwAcsEntrySecRwLtStLgrstUpwdPos_Val/1 -> TrgtPosSelcNo4sMd/5
  PA_KeSMSw4SLegrstOpenMdSecRwLtStLgrstUpwdDnwdPosMax_Val/1 -> TrgtPosSelcOnly4sMd2/2
  TrgtPosSelcOnly4sMd2/1 -> Data Type Conversion7/1
  PA_KeSMSw4SLegrstOpenMdSecRwLtStLgrstUpwdDnwdPos_Val/1 -> TrgtPosSelcOnly4sMd2/1
  PA_KeSMSwRecoveryMdSecRwLtStLgrstUpwdDnwdPos_Val/1 -> TrgtPosSelc/9
  StNumFlg_Is6s_read/1 -> [Is6s], TrgtPosSelcNo4sMd/1
  TrgtPosSelcOnly4sMd1/1 -> Data Type Conversion6/1
  PA_KeSMSw4sLyingMDSecRwLtStLgrstUpwdDnwdPos_Val/1 -> TrgtPosSelcOnly4sMd1/1
  PA_KeSMSw6sRecoveryMdSecRwLtStLgrstUpwdDnwdPosMin_Val/1 -> TrgtPosSelc/8
  PA_KeSMSwRecoveryMdSecRwLtStLgrstUpwdDnwdPosMax_Val/1 -> TrgtPosSelc/10
  PA_KeSMSwRecoveryMdSecRwLtStLgrstUpwdDnwdPosMin_Val/1 -> TrgtPosSelc/11
  PA_KeSMSw6sAcsEntrySecRwLtStLgrstUpwdPos_Val/1 -> TrgtPosSelcNo4sMd/2
  PA_KeSMSw4SLegrstCloseMdSecRwLtStLgrstUpwdDnwdPos_Val/1 -> TrgtPosSelcOnly4sMd/1
  TrgtPosSelc/1 -> Data Type Conversion3/1
  TrgtPosSelcOnly4sMd3/1 -> Data Type Conversion1/1
  TrgtPosSelcOnly4sMd4/1 -> Data Type Conversion/1
  PA_KeSMSw4SAcsMd22SecRwLtStLegrstUpwdDnwdPosMax_Val/1 -> TrgtPosSelcOnly4sMd3/2
  PA_KeSMSw4SAcsMd22SecRwLtStLegrstUpwdDnwdPosMin_Val/1 -> TrgtPosSelcOnly4sMd3/3
  PA_KeSMSw4SAcsMd22SecRwLtStLegrstUpwdDnwdPos_Val/1 -> TrgtPosSelcOnly4sMd3/1
  PA_KeSMSw4SAcsMd26SecRwLtStLegrstUpwdDnwdPosMax_Val/1 -> TrgtPosSelcOnly4sMd4/2
  PA_KeSMSw4SAcsMd26SecRwLtStLegrstUpwdDnwdPosMin_Val/1 -> TrgtPosSelcOnly4sMd4/3
  PA_KeSMSw4SAcsMd26SecRwLtStLegrstUpwdDnwdPos_Val/1 -> TrgtPosSelcOnly4sMd4/1
  Data Type Conversion/1 -> KeSMSw4SAcsMd26LgrstUpwdDnwdTrgtPosCalib_TrgtPosArray_write/1
  Data Type Conversion1/1 -> KeSMSw4SAcsMd22LgrstUpwdDnwdTrgtPosCalib_TrgtPosArray_write/1
  Data Type Conversion3/1 -> RecvLR2LLgrstUpwdDnwdTrgtPosCalib_TrgtPosArray_write/1
  Data Type Conversion4/1 -> EZQR2LLgrstUpwdDnwdTrgtPosCalib_TrgtPosArray_write/1
  Data Type Conversion5/1 -> EZER2LLgrstUpwdDnwdTrgtPosCalib_TrgtPosArray_write/1
  Data Type Conversion6/1 -> LyLR2LLgrstUpwdDnwdTrgtPosCalib_TrgtPosArray_write/1
  Data Type Conversion7/1 -> LgrstOpenLR2LLgrstUpwdDnwdTrgtPosCalib_TrgtPosArray_write/1
  Data Type Conversion8/1 -> LgrstCloseLR2LLgrstUpwdDnwdTrgtPosCalib_TrgtPosArray_write/1
